simulink library "PRISMA"  (R2025b)
settings: Solver=VariableStepAuto  StartTime=0.0  StopTime=10.0  RelTol=1e-3
libraries: $bdroot x116, etargetslib x30, simulink x9
(part 1 of 3)
settings Model: Creator=Scythe  LastModifiedBy=Scythe
settings OptimizationCC: ReuseModelBlockBuffer=off
settings RTWCC: GPUComputeCapability=3.5

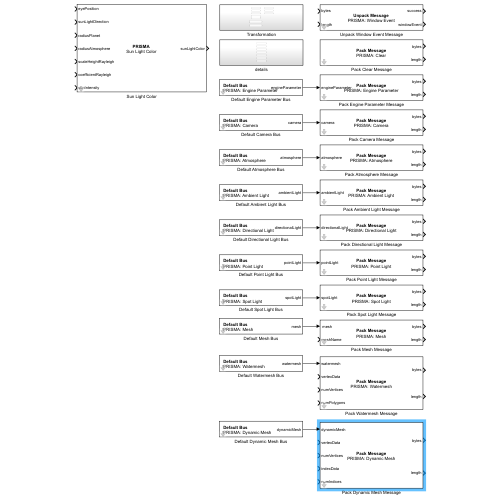
[thumbnail: Simulink's stored preview of the top-level diagram]
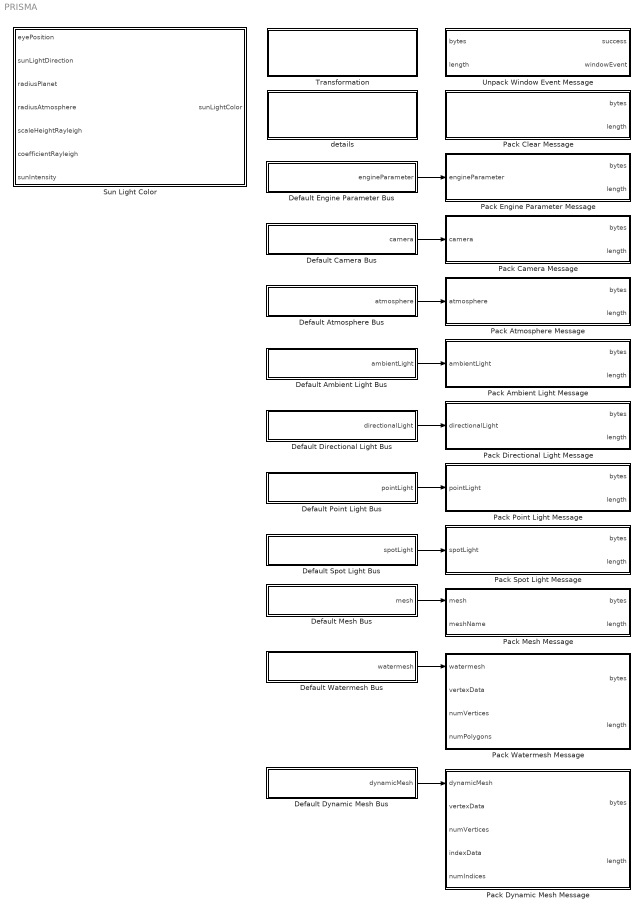
== system PRISMA ==
  Default Ambient Light Bus : Subsystem
      mask help: Create a default ambient light bus.
      mask DialogControl DescGroupVar Prompt: Default Ambient Light Bus
      mask Display:
      | text(0.05, 0.5, '{\bfDefault Bus}','horizontalAlignment','left','verticalAlignment','bottom','texmode','on');
      | text(0.05, 0.5, 'PRISMA: Ambient Light','horizontalAlignment','left','verticalAlignment','top');
  Default Atmosphere Bus : Subsystem
      mask help: Create a default atmosphere bus.
      mask DialogControl DescGroupVar Prompt: Default Atmosphere Bus
      mask Display:
      | text(0.05, 0.5, '{\bfDefault Bus}','horizontalAlignment','left','verticalAlignment','bottom','texmode','on');
      | text(0.05, 0.5, 'PRISMA: Atmosphere','horizontalAlignment','left','verticalAlignment','top');
  Default Camera Bus : Subsystem
      mask help: Create a default camera bus.
      mask DialogControl DescGroupVar Prompt: Default Camera Bus
      mask Display:
      | text(0.05, 0.5, '{\bfDefault Bus}','horizontalAlignment','left','verticalAlignment','bottom','texmode','on');
      | text(0.05, 0.5, 'PRISMA: Camera','horizontalAlignment','left','verticalAlignment','top');
  Default Directional Light Bus : Subsystem
      mask help: Create a default directional light bus.
      mask DialogControl DescGroupVar Prompt: Default Directional Light Bus
      mask Display:
      | text(0.05, 0.5, '{\bfDefault Bus}','horizontalAlignment','left','verticalAlignment','bottom','texmode','on');
      | text(0.05, 0.5, 'PRISMA: Directional Light','horizontalAlignment','left','verticalAlignment','top');
  Default Dynamic Mesh Bus : Subsystem
      mask help: Create a default dynamic mesh bus.
      mask DialogControl DescGroupVar Prompt: Default Dynamic Mesh Bus
      mask Display:
      | text(0.05, 0.5, '{\bfDefault Bus}','horizontalAlignment','left','verticalAlignment','bottom','texmode','on');
      | text(0.05, 0.5, 'PRISMA: Dynamic Mesh','horizontalAlignment','left','verticalAlignment','top');
  Default Engine Parameter Bus : Subsystem
      mask help: Create a default engine parameter bus.
      mask DialogControl DescGroupVar Prompt: Default Engine Parameter Bus
      mask Display:
      | text(0.05, 0.5, '{\bfDefault Bus}','horizontalAlignment','left','verticalAlignment','bottom','texmode','on');
      | text(0.05, 0.5, 'PRISMA: Engine Parameter','horizontalAlignment','left','verticalAlignment','top');
  Default Mesh Bus : Subsystem
      mask help: Create a default mesh bus.
      mask DialogControl DescGroupVar Prompt: Default Mesh Bus
      mask Display:
      | text(0.05, 0.5, '{\bfDefault Bus}','horizontalAlignment','left','verticalAlignment','bottom','texmode','on');
      | text(0.05, 0.5, 'PRISMA: Mesh','horizontalAlignment','left','verticalAlignment','top');
  Default Point Light Bus : Subsystem
      mask help: Create a default point light bus.
      mask DialogControl DescGroupVar Prompt: Default Point Light Bus
      mask Display:
      | text(0.05, 0.5, '{\bfDefault Bus}','horizontalAlignment','left','verticalAlignment','bottom','texmode','on');
      | text(0.05, 0.5, 'PRISMA: Point Light','horizontalAlignment','left','verticalAlignment','top');
  Default Spot Light Bus : Subsystem
      mask help: Create a default spot light bus.
      mask DialogControl DescGroupVar Prompt: Default Spot Light Bus
      mask Display:
      | text(0.05, 0.5, '{\bfDefault Bus}','horizontalAlignment','left','verticalAlignment','bottom','texmode','on');
      | text(0.05, 0.5, 'PRISMA: Spot Light','horizontalAlignment','left','verticalAlignment','top');
  Default Watermesh Bus : Subsystem
      mask help: Create a default watermesh bus.
      mask DialogControl DescGroupVar Prompt: Default Watermesh Bus
      mask Display:
      | text(0.05, 0.5, '{\bfDefault Bus}','horizontalAlignment','left','verticalAlignment','bottom','texmode','on');
      | text(0.05, 0.5, 'PRISMA: Watermesh','horizontalAlignment','left','verticalAlignment','top');
  Pack Ambient Light Message : Subsystem
      mask help: Pack an ambient light message for PRISMA.
      mask DialogControl DescGroupVar Prompt: Pack Ambient Light Message
      mask Display:
      | text(0.5, 0.5, '{\bfPack Message}','horizontalAlignment','center','verticalAlignment','bottom','texmode','on');
      | text(0.5, 0.5, 'PRISMA: Ambient Light','horizontalAlignment','center','verticalAlignment','top');
  Pack Atmosphere Message : Subsystem
      mask help: Pack an atmosphere message for PRISMA.
      mask DialogControl DescGroupVar Prompt: Pack Atmosphere Message
      mask Display:
      | text(0.5, 0.5, '{\bfPack Message}','horizontalAlignment','center','verticalAlignment','bottom','texmode','on');
      | text(0.5, 0.5, 'PRISMA: Atmosphere','horizontalAlignment','center','verticalAlignment','top');
  Pack Camera Message : Subsystem
      mask help: Pack a camera message for PRISMA.
      mask DialogControl DescGroupVar Prompt: Pack Camera Message
      mask Display:
      | text(0.5, 0.5, '{\bfPack Message}','horizontalAlignment','center','verticalAlignment','bottom','texmode','on');
      | text(0.5, 0.5, 'PRISMA: Camera','horizontalAlignment','center','verticalAlignment','top');
  Pack Clear Message : Subsystem
      mask help: Pack a clear message for PRISMA.
      mask DialogControl DescGroupVar Prompt: Pack Clear Message
      mask Display:
      | text(0.5, 0.5, '{\bfPack Message}','horizontalAlignment','center','verticalAlignment','bottom','texmode','on');
      | text(0.5, 0.5, 'PRISMA: Clear','horizontalAlignment','center','verticalAlignment','top');
  Pack Directional Light Message : Subsystem
      mask help: Pack a directional light message for PRISMA.
      mask DialogControl DescGroupVar Prompt: Pack Directional Light Message
      mask Display:
      | text(0.5, 0.5, '{\bfPack Message}','horizontalAlignment','center','verticalAlignment','bottom','texmode','on');
      | text(0.5, 0.5, 'PRISMA: Directional Light','horizontalAlignment','center','verticalAlignment','top');
  Pack Dynamic Mesh Message : Subsystem
      mask help: Pack a dynamic mesh message for PRISMA.
      mask DialogControl DescGroupVar Prompt: Pack Dynamic Mesh Message
      mask Display:
      | text(0.5, 0.5, '{\bfPack Message}','horizontalAlignment','center','verticalAlignment','bottom','texmode','on');
      | text(0.5, 0.5, 'PRISMA: Dynamic Mesh','horizontalAlignment','center','verticalAlignment','top');
  Pack Engine Parameter Message : Subsystem
      mask help: Pack an engine parameter message for PRISMA.
      mask DialogControl DescGroupVar Prompt: Pack Engine Parameter Message
      mask Display:
      | text(0.5, 0.5, '{\bfPack Message}','horizontalAlignment','center','verticalAlignment','bottom','texmode','on');
      | text(0.5, 0.5, 'PRISMA: Engine Parameter','horizontalAlignment','center','verticalAlignment','top');
  Pack Mesh Message : Subsystem
      mask help: Pack a mesh message for PRISMA.
      mask DialogControl DescGroupVar Prompt: Pack Mesh Message
      mask Display:
      | text(0.5, 0.5, '{\bfPack Message}','horizontalAlignment','center','verticalAlignment','bottom','texmode','on');
      | text(0.5, 0.5, 'PRISMA: Mesh','horizontalAlignment','center','verticalAlignment','top');
  Pack Point Light Message : Subsystem
      mask help: Pack a point light message for PRISMA.
      mask DialogControl DescGroupVar Prompt: Pack Point Light Message
      mask Display:
      | text(0.5, 0.5, '{\bfPack Message}','horizontalAlignment','center','verticalAlignment','bottom','texmode','on');
      | text(0.5, 0.5, 'PRISMA: Point Light','horizontalAlignment','center','verticalAlignment','top');
  Pack Spot Light Message : Subsystem
      mask help: Pack a spot light message for PRISMA.
      mask DialogControl DescGroupVar Prompt: Pack Spot Light Message
      mask Display:
      | text(0.5, 0.5, '{\bfPack Message}','horizontalAlignment','center','verticalAlignment','bottom','texmode','on');
      | text(0.5, 0.5, 'PRISMA: Spot Light','horizontalAlignment','center','verticalAlignment','top');
  Pack Watermesh Message : Subsystem
      mask help: Pack a watermesh message for PRISMA.
      mask DialogControl DescGroupVar Prompt: Pack Watermesh Message
      mask Display:
      | text(0.5, 0.5, '{\bfPack Message}','horizontalAlignment','center','verticalAlignment','bottom','texmode','on');
      | text(0.5, 0.5, 'PRISMA: Watermesh','horizontalAlignment','center','verticalAlignment','top');
  Sun Light Color : Subsystem
      mask help: Calculate the sun color based on Rayleigh scattering.
      mask DialogControl DescGroupVar Prompt: Sun Light Color
      mask Display:
      | text(0.5, 0.5, '{\bfPRISMA}','horizontalAlignment','center','verticalAlignment','bottom','texmode','on');
      | text(0.5, 0.5, 'Sun Light Color','horizontalAlignment','center','verticalAlignment','top');
  Transformation : Subsystem
  Unpack Window Event Message : Subsystem
      mask help: Unpack a window event message from PRISMA.
      mask DialogControl DescGroupVar Prompt: Unpack Window Event Message
      mask Display:
      | text(0.5, 0.5, '{\bfUnpack Message}','horizontalAlignment','center','verticalAlignment','bottom','texmode','on');
      | text(0.5, 0.5, 'PRISMA: Window Event','horizontalAlignment','center','verticalAlignment','top');
  details : Subsystem
  wires:
  Default Mesh Bus/1(mesh) -> Pack Mesh Message/1(" mesh")
  Default Ambient Light Bus/1(ambientLight) -> Pack Ambient Light Message/1(ambientLight)
  Default Atmosphere Bus/1(atmosphere) -> Pack Atmosphere Message/1(atmosphere)
  Default Camera Bus/1(camera) -> Pack Camera Message/1(camera)
  Default Directional Light Bus/1(directionalLight) -> Pack Directional Light Message/1(directionalLight)
  Default Engine Parameter Bus/1(engineParameter) -> Pack Engine Parameter Message/1(engineParameter)
  Default Point Light Bus/1(pointLight) -> Pack Point Light Message/1(pointLight)
  Default Spot Light Bus/1(spotLight) -> Pack Spot Light Message/1(spotLight)
  Default Watermesh Bus/1(watermesh) -> Pack Watermesh Message/1(watermesh)
  Default Dynamic Mesh Bus/1(dynamicMesh) -> Pack Dynamic Mesh Message/1(dynamicMesh)

== system PRISMA/Default Ambient Light Bus ==
  Constant : Constant  Value=[0;0;0]
  Signal Specification20 : SignalSpecification  OutDataTypeStr=double  Dimensions=3
  Bus Element Out : Outport  PortName=ambientLight  Element=color
  wires:
  Signal Specification20/1 -> Bus Element Out/1
  Constant/1 -> Signal Specification20/1

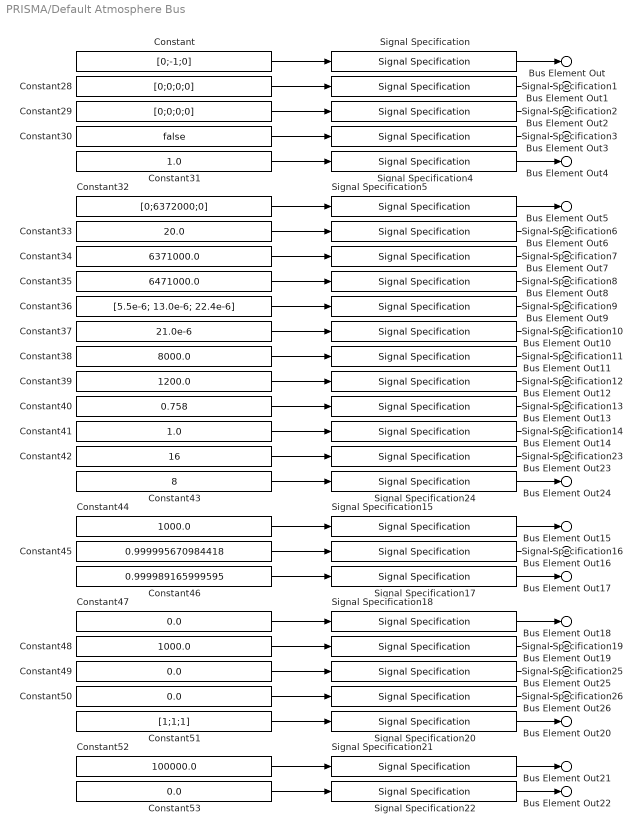
== system PRISMA/Default Atmosphere Bus ==
  Constant : Constant  Value=[0;-1;0]
  Constant28 : Constant  Value=[0;0;0;0]
  Constant29 : Constant  Value=[0;0;0;0]
  Constant30 : Constant  Value=false  OutDataTypeStr=boolean
  Constant31 : Constant  Value=1.0
  Constant32 : Constant  Value=[0;6372000;0]
  Constant33 : Constant  Value=20.0
  Constant34 : Constant  Value=6371000.0
  Constant35 : Constant  Value=6471000.0
  Constant36 : Constant  Value=[5.5e-6; 13.0e-6; 22.4e-6]
  Constant37 : Constant  Value=21.0e-6
  Constant38 : Constant  Value=8000.0
  Constant39 : Constant  Value=1200.0
  Constant40 : Constant  Value=0.758
  Constant41 : Constant  Value=1.0
  Constant42 : Constant  Value=16  OutDataTypeStr=uint8
  Constant43 : Constant  Value=8  OutDataTypeStr=uint8
  Constant44 : Constant  Value=1000.0
  Constant45 : Constant  Value=0.999995670984418
  Constant46 : Constant  Value=0.999989165999595
  Constant{47,49..50,53} (4 alike) : Constant  Value=0.0
  Constant48 : Constant  Value=1000.0
  Constant51 : Constant  Value=[1;1;1]
  Constant52 : Constant  Value=100000.0
  Signal Specification{,5,9,20} (4 alike) : SignalSpecification  OutDataTypeStr=double  Dimensions=3
  Signal Specification1 : SignalSpecification  OutDataTypeStr=double  Dimensions=4
  Signal Specification{4,6..8,10..19,21..22,25..26} (18 alike) : SignalSpecification  OutDataTypeStr=double  Dimensions=1
  Signal Specification2 : SignalSpecification  OutDataTypeStr=double  Dimensions=4
  Signal Specification23 : SignalSpecification  OutDataTypeStr=uint8  Dimensions=1
  Signal Specification24 : SignalSpecification  OutDataTypeStr=uint8  Dimensions=1
  Signal Specification3 : SignalSpecification  OutDataTypeStr=boolean  Dimensions=1
  Bus Element Out : Outport  PortName=atmosphere  Element=basicProperties.sunLightDirection
  Bus Element Out1 : Outport  PortName=atmosphere  Element=basicProperties.skyColorMix
  Bus Element Out2 : Outport  PortName=atmosphere  Element=basicProperties.sunColorMix
  Bus Element Out3 : Outport  PortName=atmosphere  Element=basicProperties.useMieForSunColor
  Bus Element Out4 : Outport  PortName=atmosphere  Element=basicProperties.sunLightStrength
  Bus Element Out5 : Outport  PortName=atmosphere  Element=atmosphericScattering.eyePosition
  Bus Element Out6 : Outport  PortName=atmosphere  Element=atmosphericScattering.sunAtmosphereIntensity
  Bus Element Out7 : Outport  PortName=atmosphere  Element=atmosphericScattering.radiusPlanet
  Bus Element Out8 : Outport  PortName=atmosphere  Element=atmosphericScattering.radiusAtmosphere
  Bus Element Out9 : Outport  PortName=atmosphere  Element=atmosphericScattering.coefficientRayleigh
  Bus Element Out10 : Outport  PortName=atmosphere  Element=atmosphericScattering.coefficientMie
  Bus Element Out11 : Outport  PortName=atmosphere  Element=atmosphericScattering.scaleHeightRayleigh
  Bus Element Out12 : Outport  PortName=atmosphere  Element=atmosphericScattering.scaleHeightMie
  Bus Element Out13 : Outport  PortName=atmosphere  Element=atmosphericScattering.scatterAmountMie
  Bus Element Out14 : Outport  PortName=atmosphere  Element=atmosphericScattering.atmosphereExposure
  Bus Element Out23 : Outport  PortName=atmosphere  Element=atmosphericScattering.numPrimaryRayTracingSteps
  Bus Element Out24 : Outport  PortName=atmosphere  Element=atmosphericScattering.numSecondaryRayTracingSteps
  Bus Element Out15 : Outport  PortName=atmosphere  Element=sunDisc.intensity
  Bus Element Out16 : Outport  PortName=atmosphere  Element=sunDisc.cosInnerCutOff
  Bus Element Out17 : Outport  PortName=atmosphere  Element=sunDisc.cosOuterCutOff
  Bus Element Out18 : Outport  PortName=atmosphere  Element=depthFog.depthBegin
  Bus Element Out19 : Outport  PortName=atmosphere  Element=depthFog.depthEnd
  Bus Element Out25 : Outport  PortName=atmosphere  Element=depthFog.densityBegin
  Bus Element Out26 : Outport  PortName=atmosphere  Element=depthFog.densityEnd
  Bus Element Out20 : Outport  PortName=atmosphere  Element=depthFog.color
  Bus Element Out21 : Outport  PortName=atmosphere  Element=sceneBlendOut.minDistance
  Bus Element Out22 : Outport  PortName=atmosphere  Element=sceneBlendOut.distanceRange
  wires:
  Constant53/1 -> Signal Specification22/1
  Constant52/1 -> Signal Specification21/1
  Constant51/1 -> Signal Specification20/1
  Constant48/1 -> Signal Specification19/1
  Constant47/1 -> Signal Specification18/1
  Constant46/1 -> Signal Specification17/1
  Constant45/1 -> Signal Specification16/1
  Constant44/1 -> Signal Specification15/1
  Constant43/1 -> Signal Specification24/1
  Constant42/1 -> Signal Specification23/1
  Constant41/1 -> Signal Specification14/1
  Constant40/1 -> Signal Specification13/1
  Constant39/1 -> Signal Specification12/1
  Constant38/1 -> Signal Specification11/1
  Constant37/1 -> Signal Specification10/1
  Constant36/1 -> Signal Specification9/1
  Constant35/1 -> Signal Specification8/1
  Constant34/1 -> Signal Specification7/1
  Constant33/1 -> Signal Specification6/1
  Constant32/1 -> Signal Specification5/1
  Constant31/1 -> Signal Specification4/1
  Constant29/1 -> Signal Specification2/1
  Constant28/1 -> Signal Specification1/1
  Signal Specification24/1 -> Bus Element Out24/1
  Signal Specification23/1 -> Bus Element Out23/1
  Signal Specification22/1 -> Bus Element Out22/1
  Signal Specification21/1 -> Bus Element Out21/1
  Signal Specification20/1 -> Bus Element Out20/1
  Signal Specification19/1 -> Bus Element Out19/1
  Signal Specification18/1 -> Bus Element Out18/1
  Signal Specification17/1 -> Bus Element Out17/1
  Signal Specification16/1 -> Bus Element Out16/1
  Signal Specification15/1 -> Bus Element Out15/1
  Signal Specification14/1 -> Bus Element Out14/1
  Signal Specification13/1 -> Bus Element Out13/1
  Signal Specification12/1 -> Bus Element Out12/1
  Signal Specification11/1 -> Bus Element Out11/1
  Signal Specification10/1 -> Bus Element Out10/1
  Signal Specification9/1 -> Bus Element Out9/1
  Signal Specification8/1 -> Bus Element Out8/1
  Signal Specification7/1 -> Bus Element Out7/1
  Signal Specification6/1 -> Bus Element Out6/1
  Signal Specification5/1 -> Bus Element Out5/1
  Signal Specification4/1 -> Bus Element Out4/1
  Constant30/1 -> Signal Specification3/1
  Signal Specification3/1 -> Bus Element Out3/1
  Signal Specification2/1 -> Bus Element Out2/1
  Signal Specification1/1 -> Bus Element Out1/1
  Constant/1 -> Signal Specification/1
  Signal Specification/1 -> Bus Element Out/1
  Signal Specification25/1 -> Bus Element Out25/1
  Signal Specification26/1 -> Bus Element Out26/1
  Constant49/1 -> Signal Specification25/1
  Constant50/1 -> Signal Specification26/1

== system PRISMA/Default Camera Bus ==
  Constant : Constant  Value=0  OutDataTypeStr=uint8
  Constant10 : Constant  Value=[0;0;0]
  Constant11 : Constant  Value=[1;0;0;0]
  Constant12 : Constant  Value=0.1
  Constant13 : Constant  Value=1000.0
  Constant14 : Constant  Value=-1.0
  Constant15 : Constant  Value=1.0
  Constant17 : Constant  Value=-1.0
  Constant18 : Constant  Value=1.0
  Constant19 : Constant  Value=deg2rad(70.0)
  Signal Specification : SignalSpecification  OutDataTypeStr=uint8  Dimensions=1
  Signal Specification1 : SignalSpecification  OutDataTypeStr=double  Dimensions=3
  Signal Specification2 : SignalSpecification  OutDataTypeStr=double  Dimensions=4
  Signal Specification{3..9} (7 alike) : SignalSpecification  OutDataTypeStr=double  Dimensions=1
  Bus Element Out : Outport  PortName=camera  Element=mode
  Bus Element Out1 : Outport  PortName=camera  Element=position
  Bus Element Out2 : Outport  PortName=camera  Element=quaternion
  Bus Element Out3 : Outport  PortName=camera  Element=clipNear
  Bus Element Out4 : Outport  PortName=camera  Element=clipFar
  Bus Element Out5 : Outport  PortName=camera  Element=orthographicLeft
  Bus Element Out6 : Outport  PortName=camera  Element=orthographicRight
  Bus Element Out7 : Outport  PortName=camera  Element=orthographicBottom
  Bus Element Out8 : Outport  PortName=camera  Element=orthographicTop
  Bus Element Out9 : Outport  PortName=camera  Element=perspectiveFieldOfView
  wires:
  Constant19/1 -> Signal Specification9/1
  Constant17/1 -> Signal Specification7/1
  Constant18/1 -> Signal Specification8/1
  Constant15/1 -> Signal Specification6/1
  Constant14/1 -> Signal Specification5/1
  Constant13/1 -> Signal Specification4/1
  Constant12/1 -> Signal Specification3/1
  Signal Specification/1 -> Bus Element Out/1
  Constant/1 -> Signal Specification/1
  Signal Specification1/1 -> Bus Element Out1/1
  Signal Specification2/1 -> Bus Element Out2/1
  Signal Specification3/1 -> Bus Element Out3/1
  Signal Specification4/1 -> Bus Element Out4/1
  Signal Specification5/1 -> Bus Element Out5/1
  Signal Specification6/1 -> Bus Element Out6/1
  Signal Specification7/1 -> Bus Element Out7/1
  Signal Specification8/1 -> Bus Element Out8/1
  Signal Specification9/1 -> Bus Element Out9/1
  Constant10/1 -> Signal Specification1/1
  Constant11/1 -> Signal Specification2/1

== system PRISMA/Default Directional Light Bus ==
  Constant : Constant  Value=[0;-1;0]
  Constant5 : Constant  Value=0  OutDataTypeStr=uint32
  Constant6 : Constant  Value=false
  Constant7 : Constant  Value=true
  Constant8 : Constant  Value=[0;0;0]
  Signal Specification1 : SignalSpecification  OutDataTypeStr=uint32  Dimensions=1
  Signal Specification2 : SignalSpecification  OutDataTypeStr=double  Dimensions=3
  Signal Specification20 : SignalSpecification  OutDataTypeStr=boolean  Dimensions=1
  Signal Specification3 : SignalSpecification  OutDataTypeStr=boolean  Dimensions=1
  Signal Specification4 : SignalSpecification  OutDataTypeStr=double  Dimensions=3
  Bus Element Out1 : Outport  PortName=directionalLight  Element=directionalLightID
  Bus Element Out : Outport  PortName=directionalLight  Element=shouldBeDeleted
  Bus Element Out3 : Outport  PortName=directionalLight  Element=visible
  Bus Element Out2 : Outport  PortName=directionalLight  Element=color
  Bus Element Out4 : Outport  PortName=directionalLight  Element=direction
  wires:
  Constant/1 -> Signal Specification4/1
  Signal Specification4/1 -> Bus Element Out4/1
  Signal Specification3/1 -> Bus Element Out3/1
  Constant7/1 -> Signal Specification3/1
  Signal Specification2/1 -> Bus Element Out2/1
  Constant8/1 -> Signal Specification2/1
  Signal Specification1/1 -> Bus Element Out1/1
  Constant5/1 -> Signal Specification1/1
  Constant6/1 -> Signal Specification20/1
  Signal Specification20/1 -> Bus Element Out/1

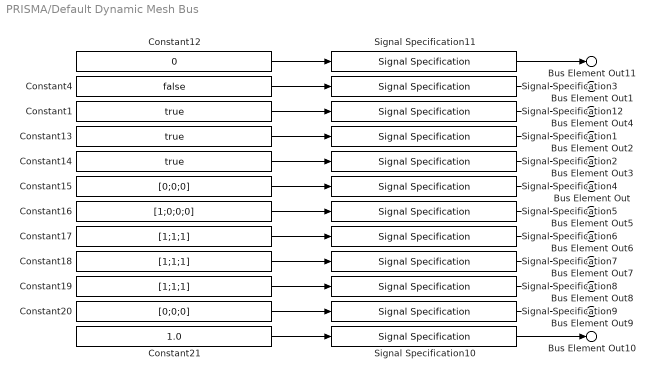
== system PRISMA/Default Dynamic Mesh Bus ==
  Constant1 : Constant  Value=true  OutDataTypeStr=boolean
  Constant12 : Constant  Value=0  OutDataTypeStr=uint32
  Constant13 : Constant  Value=true  OutDataTypeStr=boolean
  Constant14 : Constant  Value=true  OutDataTypeStr=boolean
  Constant15 : Constant  Value=[0;0;0]
  Constant16 : Constant  Value=[1;0;0;0]
  Constant17 : Constant  Value=[1;1;1]
  Constant18 : Constant  Value=[1;1;1]
  Constant19 : Constant  Value=[1;1;1]
  Constant20 : Constant  Value=[0;0;0]
  Constant21 : Constant  Value=1.0
  Constant4 : Constant  Value=false  OutDataTypeStr=boolean
  Signal Specification{1..3,12} (4 alike) : SignalSpecification  OutDataTypeStr=boolean  Dimensions=1
  Signal Specification10 : SignalSpecification  OutDataTypeStr=double  Dimensions=1
  Signal Specification11 : SignalSpecification  OutDataTypeStr=uint32  Dimensions=1
  Signal Specification{4,6..9} (5 alike) : SignalSpecification  OutDataTypeStr=double  Dimensions=3
  Signal Specification5 : SignalSpecification  OutDataTypeStr=double  Dimensions=4
  Bus Element Out11 : Outport  PortName=dynamicMesh  Element=meshID
  Bus Element Out1 : Outport  PortName=dynamicMesh  Element=shouldBeDeleted
  Bus Element Out4 : Outport  PortName=dynamicMesh  Element=updateMesh
  Bus Element Out2 : Outport  PortName=dynamicMesh  Element=visible
  Bus Element Out3 : Outport  PortName=dynamicMesh  Element=castShadow
  Bus Element Out : Outport  PortName=dynamicMesh  Element=position
  Bus Element Out5 : Outport  PortName=dynamicMesh  Element=quaternion
  Bus Element Out6 : Outport  PortName=dynamicMesh  Element=scale
  Bus Element Out7 : Outport  PortName=dynamicMesh  Element=diffuseColorMultiplier
  Bus Element Out8 : Outport  PortName=dynamicMesh  Element=specularColorMultiplier
  Bus Element Out9 : Outport  PortName=dynamicMesh  Element=emissionColorMultiplier
  Bus Element Out10 : Outport  PortName=dynamicMesh  Element=shininessMultiplier
  wires:
  Constant13/1 -> Signal Specification1/1
  Signal Specification3/1 -> Bus Element Out1/1
  Signal Specification5/1 -> Bus Element Out5/1
  Constant16/1 -> Signal Specification5/1
  Constant21/1 -> Signal Specification10/1
  Signal Specification9/1 -> Bus Element Out9/1
  Constant20/1 -> Signal Specification9/1
  Constant12/1 -> Signal Specification11/1
  Signal Specification11/1 -> Bus Element Out11/1
  Constant19/1 -> Signal Specification8/1
  Signal Specification7/1 -> Bus Element Out7/1
  Signal Specification2/1 -> Bus Element Out3/1
  Signal Specification8/1 -> Bus Element Out8/1
  Signal Specification10/1 -> Bus Element Out10/1
  Constant18/1 -> Signal Specification7/1
  Signal Specification1/1 -> Bus Element Out2/1
  Constant17/1 -> Signal Specification6/1
  Signal Specification4/1 -> Bus Element Out/1
  Signal Specification6/1 -> Bus Element Out6/1
  Constant14/1 -> Signal Specification2/1
  Constant15/1 -> Signal Specification4/1
  Constant4/1 -> Signal Specification3/1
  Signal Specification12/1 -> Bus Element Out4/1
  Constant1/1 -> Signal Specification12/1

== system PRISMA/Default Engine Parameter Bus ==
  Constant : Constant  Value=2.0
  Constant13 : Constant  Value=0.025
  Constant{14..16,22} (4 alike) : Constant  Value=1.0
  Constant17 : Constant  Value=0.1
  Constant18 : Constant  Value=2.2
  Constant19 : Constant  Value=0.5 / 255.0
  Constant20 : Constant  Value=0.0001
  Constant21 : Constant  Value=0.005
  Constant23 : Constant  Value=0.42
  Signal Specification{1..12} (12 alike) : SignalSpecification  OutDataTypeStr=double  Dimensions=1
  Bus Element Out3 : Outport  PortName=engineParameter  Element=ambientOcclusionRadius
  Bus Element Out1 : Outport  PortName=engineParameter  Element=ambientOcclusionBias
  Bus Element Out2 : Outport  PortName=engineParameter  Element=ambientOcclusionEnhance
  Bus Element Out4 : Outport  PortName=engineParameter  Element=removeShadowOnWater
  Bus Element Out5 : Outport  PortName=engineParameter  Element=bloomBrightnessThreshold
  Bus Element Out6 : Outport  PortName=engineParameter  Element=bloomStrength
  Bus Element Out7 : Outport  PortName=engineParameter  Element=gamma
  Bus Element Out8 : Outport  PortName=engineParameter  Element=ditheringNoiseGranularity
  Bus Element Out9 : Outport  PortName=engineParameter  Element=shadowBiasMin
  Bus Element Out10 : Outport  PortName=engineParameter  Element=shadowBiasMax
  Bus Element Out11 : Outport  PortName=engineParameter  Element=exposure
  Bus Element Out12 : Outport  PortName=engineParameter  Element=toneMappingStrength
  wires:
  Constant23/1 -> Signal Specification12/1
  Signal Specification12/1 -> Bus Element Out12/1
  Signal Specification11/1 -> Bus Element Out11/1
  Constant22/1 -> Signal Specification11/1
  Constant21/1 -> Signal Specification10/1
  Signal Specification10/1 -> Bus Element Out10/1
  Signal Specification9/1 -> Bus Element Out9/1
  Constant20/1 -> Signal Specification9/1
  Constant19/1 -> Signal Specification8/1
  Signal Specification8/1 -> Bus Element Out8/1
  Signal Specification7/1 -> Bus Element Out7/1
  Constant18/1 -> Signal Specification7/1
  Constant17/1 -> Signal Specification6/1
  Signal Specification6/1 -> Bus Element Out6/1
  Signal Specification5/1 -> Bus Element Out5/1
  Constant16/1 -> Signal Specification5/1
  Constant15/1 -> Signal Specification4/1
  Signal Specification4/1 -> Bus Element Out4/1
  Signal Specification2/1 -> Bus Element Out2/1
  Constant14/1 -> Signal Specification2/1
  Constant13/1 -> Signal Specification1/1
  Signal Specification1/1 -> Bus Element Out1/1
  Signal Specification3/1 -> Bus Element Out3/1
  Constant/1 -> Signal Specification3/1

== system PRISMA/Default Mesh Bus ==
  Constant12 : Constant  Value=0  OutDataTypeStr=uint32
  Constant13 : Constant  Value=true  OutDataTypeStr=boolean
  Constant14 : Constant  Value=true  OutDataTypeStr=boolean
  Constant15 : Constant  Value=[0;0;0]
  Constant16 : Constant  Value=[1;0;0;0]
  Constant17 : Constant  Value=[1;1;1]
  Constant18 : Constant  Value=[1;1;1]
  Constant19 : Constant  Value=[1;1;1]
  Constant20 : Constant  Value=[0;0;0]
  Constant21 : Constant  Value=1.0
  Constant4 : Constant  Value=false  OutDataTypeStr=boolean
  Signal Specification1 : SignalSpecification  OutDataTypeStr=boolean  Dimensions=1
  Signal Specification10 : SignalSpecification  OutDataTypeStr=double  Dimensions=1
  Signal Specification11 : SignalSpecification  OutDataTypeStr=uint32  Dimensions=1
  Signal Specification2 : SignalSpecification  OutDataTypeStr=boolean  Dimensions=1
  Signal Specification3 : SignalSpecification  OutDataTypeStr=boolean  Dimensions=1
  Signal Specification{4,6..9} (5 alike) : SignalSpecification  OutDataTypeStr=double  Dimensions=3
  Signal Specification5 : SignalSpecification  OutDataTypeStr=double  Dimensions=4
  Bus Element Out11 : Outport  PortName=mesh  Element=meshID
  Bus Element Out1 : Outport  PortName=mesh  Element=shouldBeDeleted
  Bus Element Out2 : Outport  PortName=mesh  Element=visible
  Bus Element Out3 : Outport  PortName=mesh  Element=castShadow
  Bus Element Out : Outport  PortName=mesh  Element=position
  Bus Element Out5 : Outport  PortName=mesh  Element=quaternion
  Bus Element Out6 : Outport  PortName=mesh  Element=scale
  Bus Element Out7 : Outport  PortName=mesh  Element=diffuseColorMultiplier
  Bus Element Out8 : Outport  PortName=mesh  Element=specularColorMultiplier
  Bus Element Out9 : Outport  PortName=mesh  Element=emissionColorMultiplier
  Bus Element Out10 : Outport  PortName=mesh  Element=shininessMultiplier
  wires:
  Signal Specification11/1 -> Bus Element Out11/1
  Constant12/1 -> Signal Specification11/1
  Signal Specification10/1 -> Bus Element Out10/1
  Constant21/1 -> Signal Specification10/1
  Constant20/1 -> Signal Specification9/1
  Signal Specification9/1 -> Bus Element Out9/1
  Constant19/1 -> Signal Specification8/1
  Signal Specification8/1 -> Bus Element Out8/1
  Signal Specification7/1 -> Bus Element Out7/1
  Constant18/1 -> Signal Specification7/1
  Constant17/1 -> Signal Specification6/1
  Signal Specification6/1 -> Bus Element Out6/1
  Signal Specification5/1 -> Bus Element Out5/1
  Constant16/1 -> Signal Specification5/1
  Signal Specification2/1 -> Bus Element Out3/1
  Constant14/1 -> Signal Specification2/1
  Constant13/1 -> Signal Specification1/1
  Signal Specification1/1 -> Bus Element Out2/1
  Signal Specification3/1 -> Bus Element Out1/1
  Constant4/1 -> Signal Specification3/1
  Constant15/1 -> Signal Specification4/1
  Signal Specification4/1 -> Bus Element Out/1

== system PRISMA/Default Point Light Bus ==
  Constant10 : Constant  Value=[0;0;0]
  Constant11 : Constant  Value=[0;0;0]
  Constant12 : Constant  Value=0.0
  Constant13 : Constant  Value=0.0
  Constant7 : Constant  Value=0  OutDataTypeStr=uint32
  Constant8 : Constant  Value=false  OutDataTypeStr=boolean
  Constant9 : Constant  Value=true  OutDataTypeStr=boolean
  Signal Specification1 : SignalSpecification  OutDataTypeStr=uint32  Dimensions=1
  Signal Specification2 : SignalSpecification  OutDataTypeStr=double  Dimensions=3
  Signal Specification20 : SignalSpecification  OutDataTypeStr=boolean  Dimensions=1
  Signal Specification3 : SignalSpecification  OutDataTypeStr=boolean  Dimensions=1
  Signal Specification4 : SignalSpecification  OutDataTypeStr=double  Dimensions=3
  Signal Specification5 : SignalSpecification  OutDataTypeStr=double  Dimensions=1
  Signal Specification6 : SignalSpecification  OutDataTypeStr=double  Dimensions=1
  Bus Element Out1 : Outport  PortName=pointLight  Element=pointLightID
  Bus Element Out : Outport  PortName=pointLight  Element=shouldBeDeleted
  Bus Element Out3 : Outport  PortName=pointLight  Element=visible
  Bus Element Out2 : Outport  PortName=pointLight  Element=color
  Bus Element Out4 : Outport  PortName=pointLight  Element=position
  Bus Element Out5 : Outport  PortName=pointLight  Element=quadraticFalloff
  Bus Element Out6 : Outport  PortName=pointLight  Element=invRadiusPow4
  wires:
  Signal Specification6/1 -> Bus Element Out6/1
  Constant13/1 -> Signal Specification6/1
  Constant12/1 -> Signal Specification5/1
  Signal Specification5/1 -> Bus Element Out5/1
  Signal Specification20/1 -> Bus Element Out/1
  Constant8/1 -> Signal Specification20/1
  Constant7/1 -> Signal Specification1/1
  Signal Specification1/1 -> Bus Element Out1/1
  Constant10/1 -> Signal Specification2/1
  Signal Specification2/1 -> Bus Element Out2/1
  Constant9/1 -> Signal Specification3/1
  Signal Specification3/1 -> Bus Element Out3/1
  Signal Specification4/1 -> Bus Element Out4/1
  Constant11/1 -> Signal Specification4/1

== system PRISMA/Default Spot Light Bus ==
  Constant10 : Constant  Value=[0;0;0]
  Constant11 : Constant  Value=[0;0;0]
  Constant12 : Constant  Value=[0;-1;0]
  Constant13 : Constant  Value=0  OutDataTypeStr=uint32
  Constant14 : Constant  Value=false  OutDataTypeStr=boolean
  Constant15 : Constant  Value=true  OutDataTypeStr=boolean
  Constant16 : Constant  Value=0.0
  Constant17 : Constant  Value=0.0
  Constant18 : Constant  Value=0.5
  Constant19 : Constant  Value=0.5
  Signal Specification1 : SignalSpecification  OutDataTypeStr=uint32  Dimensions=1
  Signal Specification2 : SignalSpecification  OutDataTypeStr=double  Dimensions=3
  Signal Specification20 : SignalSpecification  OutDataTypeStr=boolean  Dimensions=1
  Signal Specification3 : SignalSpecification  OutDataTypeStr=boolean  Dimensions=1
  Signal Specification4 : SignalSpecification  OutDataTypeStr=double  Dimensions=3
  Signal Specification5 : SignalSpecification  OutDataTypeStr=double  Dimensions=3
  Signal Specification{6..9} (4 alike) : SignalSpecification  OutDataTypeStr=double  Dimensions=1
  Bus Element Out1 : Outport  PortName=spotLight  Element=spotLightID
  Bus Element Out : Outport  PortName=spotLight  Element=shouldBeDeleted
  Bus Element Out3 : Outport  PortName=spotLight  Element=visible
  Bus Element Out2 : Outport  PortName=spotLight  Element=color
  Bus Element Out4 : Outport  PortName=spotLight  Element=position
  Bus Element Out7 : Outport  PortName=spotLight  Element=direction
  Bus Element Out5 : Outport  PortName=spotLight  Element=quadraticFalloff
  Bus Element Out6 : Outport  PortName=spotLight  Element=invRadiusPow4
  Bus Element Out8 : Outport  PortName=spotLight  Element=cosInnerCutOffAngle
  Bus Element Out9 : Outport  PortName=spotLight  Element=cosOuterCutOffAngle
  wires:
  Constant19/1 -> Signal Specification9/1
  Signal Specification9/1 -> Bus Element Out9/1
  Signal Specification8/1 -> Bus Element Out8/1
  Constant18/1 -> Signal Specification8/1
  Signal Specification5/1 -> Bus Element Out7/1
  Constant12/1 -> Signal Specification5/1
  Constant10/1 -> Signal Specification4/1
  Signal Specification4/1 -> Bus Element Out4/1
  Signal Specification3/1 -> Bus Element Out3/1
  Constant15/1 -> Signal Specification3/1
  Signal Specification2/1 -> Bus Element Out2/1
  Constant11/1 -> Signal Specification2/1
  Signal Specification1/1 -> Bus Element Out1/1
  Constant13/1 -> Signal Specification1/1
  Constant14/1 -> Signal Specification20/1
  Signal Specification20/1 -> Bus Element Out/1
  Signal Specification6/1 -> Bus Element Out5/1
  Constant16/1 -> Signal Specification6/1
  Constant17/1 -> Signal Specification7/1
  Signal Specification7/1 -> Bus Element Out6/1

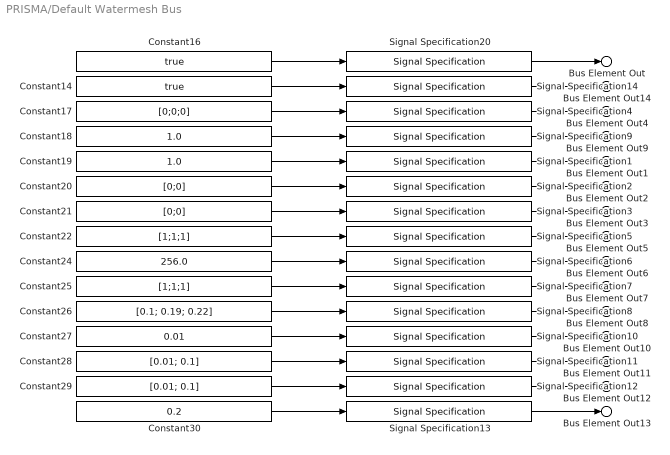
== system PRISMA/Default Watermesh Bus ==
  Constant14 : Constant  Value=true  OutDataTypeStr=boolean
  Constant16 : Constant  Value=true  OutDataTypeStr=boolean
  Constant17 : Constant  Value=[0;0;0]
  Constant18 : Constant  Value=1.0
  Constant19 : Constant  Value=1.0
  Constant20 : Constant  Value=[0;0]
  Constant21 : Constant  Value=[0;0]
  Constant22 : Constant  Value=[1;1;1]
  Constant24 : Constant  Value=256.0
  Constant25 : Constant  Value=[1;1;1]
  Constant26 : Constant  Value=[0.1; 0.19; 0.22]
  Constant27 : Constant  Value=0.01
  Constant28 : Constant  Value=[0.01; 0.1]
  Constant29 : Constant  Value=[0.01; 0.1]
  Constant30 : Constant  Value=0.2
  Signal Specification{1,6,9..10,13} (5 alike) : SignalSpecification  OutDataTypeStr=double  Dimensions=1
  Signal Specification{2..3,11..12} (4 alike) : SignalSpecification  OutDataTypeStr=double  Dimensions=2
  Signal Specification14 : SignalSpecification  OutDataTypeStr=boolean  Dimensions=1
  Signal Specification20 : SignalSpecification  OutDataTypeStr=boolean  Dimensions=1
  Signal Specification{4..5,7..8} (4 alike) : SignalSpecification  OutDataTypeStr=double  Dimensions=3
  Bus Element Out : Outport  PortName=watermesh  Element=updateMesh
  Bus Element Out14 : Outport  PortName=watermesh  Element=visible
  Bus Element Out4 : Outport  PortName=watermesh  Element=position
  Bus Element Out9 : Outport  PortName=watermesh  Element=textureCoordinateScaling1
  Bus Element Out1 : Outport  PortName=watermesh  Element=textureCoordinateScaling2
  Bus Element Out2 : Outport  PortName=watermesh  Element=textureCoordinateAnimation1
  Bus Element Out3 : Outport  PortName=watermesh  Element=textureCoordinateAnimation2
  Bus Element Out5 : Outport  PortName=watermesh  Element=specularColor
  Bus Element Out6 : Outport  PortName=watermesh  Element=shininess
  Bus Element Out7 : Outport  PortName=watermesh  Element=reflectionColorMultiplier
  Bus Element Out8 : Outport  PortName=watermesh  Element=refractionColorMultiplier
  Bus Element Out10 : Outport  PortName=watermesh  Element=clippingPlaneOffset
  Bus Element Out11 : Outport  PortName=watermesh  Element=strengthDuDvNormal1
  Bus Element Out12 : Outport  PortName=watermesh  Element=strengthDuDvNormal2
  Bus Element Out13 : Outport  PortName=watermesh  Element=distortionWaterDepthScale
  wires:
  Constant30/1 -> Signal Specification13/1
  Signal Specification13/1 -> Bus Element Out13/1
  Constant29/1 -> Signal Specification12/1
  Signal Specification12/1 -> Bus Element Out12/1
  Signal Specification11/1 -> Bus Element Out11/1
  Constant28/1 -> Signal Specification11/1
  Signal Specification10/1 -> Bus Element Out10/1
  Constant27/1 -> Signal Specification10/1
  Constant26/1 -> Signal Specification8/1
  Signal Specification8/1 -> Bus Element Out8/1
  Signal Specification7/1 -> Bus Element Out7/1
  Constant25/1 -> Signal Specification7/1
  Constant24/1 -> Signal Specification6/1
  Signal Specification6/1 -> Bus Element Out6/1
  Constant22/1 -> Signal Specification5/1
  Signal Specification5/1 -> Bus Element Out5/1
  Signal Specification3/1 -> Bus Element Out3/1
  Constant21/1 -> Signal Specification3/1
  Constant20/1 -> Signal Specification2/1
  Signal Specification2/1 -> Bus Element Out2/1
  Constant19/1 -> Signal Specification1/1
  Signal Specification1/1 -> Bus Element Out1/1
  Signal Specification20/1 -> Bus Element Out/1
  Constant16/1 -> Signal Specification20/1
  Signal Specification4/1 -> Bus Element Out4/1
  Constant17/1 -> Signal Specification4/1
  Signal Specification9/1 -> Bus Element Out9/1
  Constant18/1 -> Signal Specification9/1
  Constant14/1 -> Signal Specification14/1
  Signal Specification14/1 -> Bus Element Out14/1

== system PRISMA/Pack Ambient Light Message ==
  Bus Element In : Inport  PortName=ambientLight  Element=color
  Byte Pack : etargetslib/Byte Pack  datatypes={'single','single','single'}  byteAlign=1
  Data Type Conversion : DataTypeConversion  OutDataTypeStr=single  SaturateOnIntegerOverflow=off  RndMeth=Floor
  Demux : Demux  Outputs=3
  PRISMA Message Type1 : $bdroot/details/PRISMA Message Type  messageType=Ambient Light
  Swap Float Native To Network : $bdroot/details/Swap Float Native To Network
  Vector Concatenate : Concatenate
  Width : Width  DataType=int32
  bytes : Outport  OutDataTypeStr=uint8
  length : Outport  Port=2  OutDataTypeStr=int32  PortDimensions=1
  wires:
  Bus Element In/1 -> Data Type Conversion/1
  Width/1 -> length/1
  Vector Concatenate/1 -> bytes/1, Width/1
  Byte Pack/1 -> Vector Concatenate/2
  PRISMA Message Type1/1 -> Vector Concatenate/1
  Data Type Conversion/1 -> Swap Float Native To Network/1
  Demux/1 -> Byte Pack/1
  Demux/2 -> Byte Pack/2
  Demux/3 -> Byte Pack/3
  Swap Float Native To Network/1 -> Demux/1

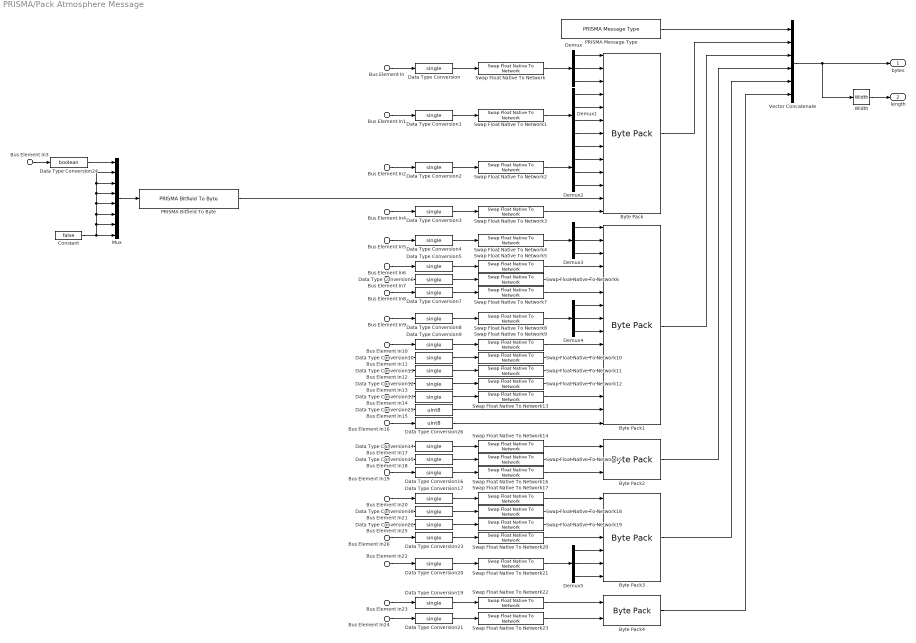
== system PRISMA/Pack Atmosphere Message ==
  Bus Element In : Inport  PortName=atmosphere  Element=basicProperties.sunLightDirection
  Bus Element In1 : Inport  PortName=atmosphere  Element=basicProperties.skyColorMix
  Bus Element In2 : Inport  PortName=atmosphere  Element=basicProperties.sunColorMix
  Bus Element In3 : Inport  PortName=atmosphere  Element=basicProperties.useMieForSunColor
  Bus Element In4 : Inport  PortName=atmosphere  Element=basicProperties.sunLightStrength
  Bus Element In5 : Inport  PortName=atmosphere  Element=atmosphericScattering.eyePosition
  Bus Element In6 : Inport  PortName=atmosphere  Element=atmosphericScattering.sunAtmosphereIntensity
  Bus Element In7 : Inport  PortName=atmosphere  Element=atmosphericScattering.radiusPlanet
  Bus Element In8 : Inport  PortName=atmosphere  Element=atmosphericScattering.radiusAtmosphere
  Bus Element In9 : Inport  PortName=atmosphere  Element=atmosphericScattering.coefficientRayleigh
  Bus Element In10 : Inport  PortName=atmosphere  Element=atmosphericScattering.coefficientMie
  Bus Element In11 : Inport  PortName=atmosphere  Element=atmosphericScattering.scaleHeightRayleigh
  Bus Element In12 : Inport  PortName=atmosphere  Element=atmosphericScattering.scaleHeightMie
  Bus Element In13 : Inport  PortName=atmosphere  Element=atmosphericScattering.scatterAmountMie
  Bus Element In14 : Inport  PortName=atmosphere  Element=atmosphericScattering.atmosphereExposure
  Bus Element In15 : Inport  PortName=atmosphere  Element=atmosphericScattering.numPrimaryRayTracingSteps
  Bus Element In16 : Inport  PortName=atmosphere  Element=atmosphericScattering.numSecondaryRayTracingSteps
  Bus Element In17 : Inport  PortName=atmosphere  Element=sunDisc.intensity
  Bus Element In18 : Inport  PortName=atmosphere  Element=sunDisc.cosInnerCutOff
  Bus Element In19 : Inport  PortName=atmosphere  Element=sunDisc.cosOuterCutOff
  Bus Element In20 : Inport  PortName=atmosphere  Element=depthFog.depthBegin
  Bus Element In21 : Inport  PortName=atmosphere  Element=depthFog.depthEnd
  Bus Element In22 : Inport  PortName=atmosphere  Element=depthFog.color
  Bus Element In25 : Inport  PortName=atmosphere  Element=depthFog.densityBegin
  Bus Element In26 : Inport  PortName=atmosphere  Element=depthFog.densityEnd
  Bus Element In23 : Inport  PortName=atmosphere  Element=sceneBlendOut.minDistance
  Bus Element In24 : Inport  PortName=atmosphere  Element=sceneBlendOut.distanceRange
  Byte Pack : etargetslib/Byte Pack  datatypes={'single','single','single','single','single','single','single','single','single','single','single','uint8','single'}  byteAlign=1
  Byte Pack1 : etargetslib/Byte Pack  datatypes={'single','single','single','single','single','single','single','single','single','single','single','single','single','single','uint8','uint8'}  byteAlign=1
  Byte Pack2 : etargetslib/Byte Pack  datatypes={'single','single','single'}  byteAlign=1
  Byte Pack3 : etargetslib/Byte Pack  datatypes={'single','single','single','single','single','single','single'}  byteAlign=1
  Byte Pack4 : etargetslib/Byte Pack  datatypes={'single','single'}  byteAlign=1
  Constant : Constant  Value=false  OutDataTypeStr=boolean
  Data Type Conversion{,1..23} (24 alike) : DataTypeConversion  OutDataTypeStr=single  SaturateOnIntegerOverflow=off  RndMeth=Floor
  Data Type Conversion24 : DataTypeConversion  OutDataTypeStr=boolean  SaturateOnIntegerOverflow=off  RndMeth=Floor
  Data Type Conversion25 : DataTypeConversion  OutDataTypeStr=uint8  SaturateOnIntegerOverflow=off  RndMeth=Floor
  Data Type Conversion26 : DataTypeConversion  OutDataTypeStr=uint8  SaturateOnIntegerOverflow=off  RndMeth=Floor
  Demux{,3..5} (4 alike) : Demux  Outputs=3
  Demux1 : Demux
  Demux2 : Demux
  Mux : Mux  Inputs=8
  PRISMA Bitfield To Byte : $bdroot/details/PRISMA Bitfield To Byte
  PRISMA Message Type : $bdroot/details/PRISMA Message Type  messageType=Atmosphere
  Swap Float Native To Network{,1..23} (24 alike) : $bdroot/details/Swap Float Native To Network
  Vector Concatenate : Concatenate  NumInputs=6
  Width : Width  DataType=int32
  bytes : Outport  OutDataTypeStr=uint8
  length : Outport  Port=2  OutDataTypeStr=int32  PortDimensions=1
  wires:
  Bus Element In24/1 -> Data Type Conversion21/1
  Data Type Conversion21/1 -> Swap Float Native To Network23/1
  Bus Element In23/1 -> Data Type Conversion19/1
  Bus Element In22/1 -> Data Type Conversion20/1
  Bus Element In21/1 -> Data Type Conversion18/1
  Bus Element In20/1 -> Data Type Conversion17/1
  Bus Element In19/1 -> Data Type Conversion16/1
  Bus Element In18/1 -> Data Type Conversion15/1
  Bus Element In17/1 -> Data Type Conversion14/1
  Bus Element In16/1 -> Data Type Conversion26/1
  Bus Element In15/1 -> Data Type Conversion25/1
  Bus Element In14/1 -> Data Type Conversion13/1
  Bus Element In13/1 -> Data Type Conversion12/1
  Bus Element In12/1 -> Data Type Conversion11/1
  Bus Element In11/1 -> Data Type Conversion10/1
  Bus Element In10/1 -> Data Type Conversion9/1
  Bus Element In9/1 -> Data Type Conversion8/1
  Bus Element In8/1 -> Data Type Conversion7/1
  Bus Element In7/1 -> Data Type Conversion6/1
  Bus Element In6/1 -> Data Type Conversion5/1
  Bus Element In5/1 -> Data Type Conversion4/1
  Bus Element In4/1 -> Data Type Conversion3/1
  Bus Element In2/1 -> Data Type Conversion2/1
  Bus Element In1/1 -> Data Type Conversion1/1
  Bus Element In/1 -> Data Type Conversion/1
  Vector Concatenate/1 -> bytes/1, Width/1
  Byte Pack4/1 -> Vector Concatenate/6
  Byte Pack3/1 -> Vector Concatenate/5
  Byte Pack2/1 -> Vector Concatenate/4
  Byte Pack1/1 -> Vector Concatenate/3
  Byte Pack/1 -> Vector Concatenate/2
  Data Type Conversion19/1 -> Swap Float Native To Network22/1
  Data Type Conversion20/1 -> Swap Float Native To Network21/1
  Data Type Conversion18/1 -> Swap Float Native To Network18/1
  Data Type Conversion17/1 -> Swap Float Native To Network17/1
  Data Type Conversion16/1 -> Swap Float Native To Network16/1
  Data Type Conversion15/1 -> Swap Float Native To Network15/1
  Data Type Conversion14/1 -> Swap Float Native To Network14/1
  Data Type Conversion13/1 -> Swap Float Native To Network13/1
  Data Type Conversion12/1 -> Swap Float Native To Network12/1
  Data Type Conversion11/1 -> Swap Float Native To Network11/1
  Data Type Conversion10/1 -> Swap Float Native To Network10/1
  Data Type Conversion9/1 -> Swap Float Native To Network9/1
  Demux4/3 -> Byte Pack1/9
  Demux4/2 -> Byte Pack1/8
  Demux4/1 -> Byte Pack1/7
  Data Type Conversion8/1 -> Swap Float Native To Network8/1
  Data Type Conversion7/1 -> Swap Float Native To Network7/1
  Data Type Conversion6/1 -> Swap Float Native To Network6/1
  Data Type Conversion5/1 -> Swap Float Native To Network5/1
  Data Type Conversion4/1 -> Swap Float Native To Network4/1
  Demux3/1 -> Byte Pack1/1
  Demux3/2 -> Byte Pack1/2
  Demux3/3 -> Byte Pack1/3
  PRISMA Bitfield To Byte/1 -> Byte Pack/12
  Mux/1 -> PRISMA Bitfield To Byte/1
  Constant/1 -> Mux/8, Mux/2, Mux/3, Mux/4, Mux/5, Mux/6, Mux/7
  Bus Element In3/1 -> Data Type Conversion24/1
  Data Type Conversion3/1 -> Swap Float Native To Network3/1
  Data Type Conversion2/1 -> Swap Float Native To Network2/1
  Demux2/4 -> Byte Pack/11
  Demux2/3 -> Byte Pack/10
  Demux2/2 -> Byte Pack/9
  Demux2/1 -> Byte Pack/8
  Data Type Conversion1/1 -> Swap Float Native To Network1/1
  Demux1/4 -> Byte Pack/7
  Demux1/3 -> Byte Pack/6
  Demux1/2 -> Byte Pack/5
  Demux1/1 -> Byte Pack/4
  Demux/3 -> Byte Pack/3
  Demux/2 -> Byte Pack/2
  Demux/1 -> Byte Pack/1
  Data Type Conversion/1 -> Swap Float Native To Network/1
  PRISMA Message Type/1 -> Vector Concatenate/1
  Width/1 -> length/1
  Data Type Conversion22/1 -> Swap Float Native To Network19/1
  Data Type Conversion23/1 -> Swap Float Native To Network20/1
  Bus Element In25/1 -> Data Type Conversion22/1
  Bus Element In26/1 -> Data Type Conversion23/1
  Demux5/1 -> Byte Pack3/5
  Demux5/2 -> Byte Pack3/6
  Demux5/3 -> Byte Pack3/7
  Data Type Conversion24/1 -> Mux/1
  Data Type Conversion25/1 -> Byte Pack1/15
  Data Type Conversion26/1 -> Byte Pack1/16
  Swap Float Native To Network/1 -> Demux/1
  Swap Float Native To Network1/1 -> Demux1/1
  Swap Float Native To Network2/1 -> Demux2/1
  Swap Float Native To Network3/1 -> Byte Pack/13
  Swap Float Native To Network4/1 -> Demux3/1
  Swap Float Native To Network5/1 -> Byte Pack1/4
  Swap Float Native To Network6/1 -> Byte Pack1/5
  Swap Float Native To Network7/1 -> Byte Pack1/6
  Swap Float Native To Network8/1 -> Demux4/1
  Swap Float Native To Network9/1 -> Byte Pack1/10
  Swap Float Native To Network10/1 -> Byte Pack1/11
  Swap Float Native To Network11/1 -> Byte Pack1/12
  Swap Float Native To Network12/1 -> Byte Pack1/13
  Swap Float Native To Network13/1 -> Byte Pack1/14
  Swap Float Native To Network14/1 -> Byte Pack2/1
  Swap Float Native To Network15/1 -> Byte Pack2/2
  Swap Float Native To Network16/1 -> Byte Pack2/3
  Swap Float Native To Network17/1 -> Byte Pack3/1
  Swap Float Native To Network18/1 -> Byte Pack3/2
  Swap Float Native To Network19/1 -> Byte Pack3/3
  Swap Float Native To Network20/1 -> Byte Pack3/4
  Swap Float Native To Network21/1 -> Demux5/1
  Swap Float Native To Network22/1 -> Byte Pack4/1
  Swap Float Native To Network23/1 -> Byte Pack4/2
